simulink model "extractLocalMap"  (R2024a)
settings: Solver=FixedStepAuto  StartTime=0.0  StopTime=10.0  RelTol=1e-3
settings Model: Creator=cstabile  LastModifiedBy=cstabile
settings SFSimCC: SimTargetLang=C++

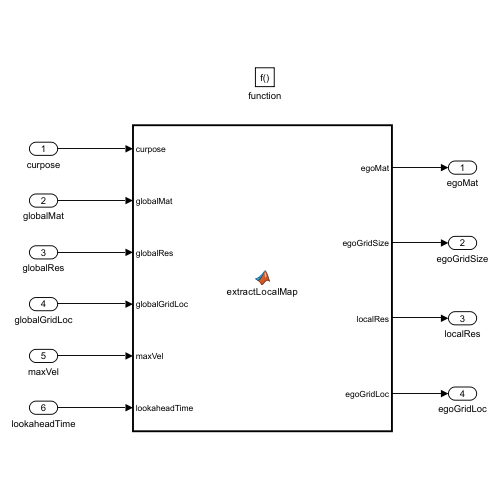
[thumbnail: Simulink's stored preview of the top-level diagram]
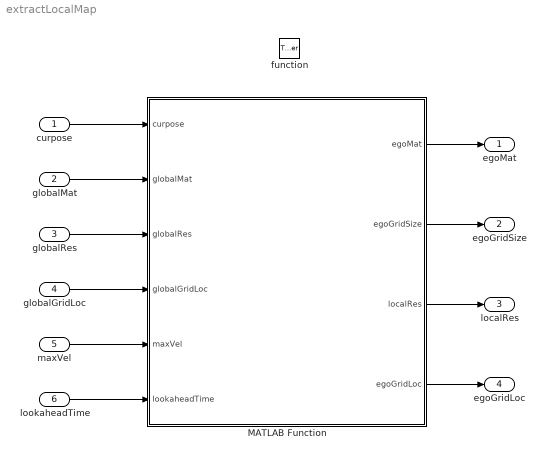
== system extractLocalMap ==
  curpose : Inport  PortDimensions=[1 3]
  globalMat : Inport  Port=2  OutDataTypeStr=boolean  PortDimensions=[1201 1201]
  globalRes : Inport  Port=3
  globalGridLoc : Inport  Port=4  PortDimensions=[1 2]
  maxVel : Inport  Port=5
  lookaheadTime : Inport  Port=6
  function : TriggerPort  TriggerType=function-call  VariantControl=(inherit)
  MATLAB Function : MATLAB Function  TreatAsAtomicUnit=on
  egoMat : Outport
  egoGridSize : Outport  Port=2
  localRes : Outport  Port=3
  egoGridLoc : Outport  Port=4
  wires:
  globalRes/1 -> MATLAB Function/3(globalRes)
  curpose/1 -> MATLAB Function/1(curpose)
  globalGridLoc/1 -> MATLAB Function/4(globalGridLoc)
  MATLAB Function/1(egoMat) -> egoMat/1
  globalMat/1 -> MATLAB Function/2(globalMat)
  maxVel/1 -> MATLAB Function/5(maxVel)
  lookaheadTime/1 -> MATLAB Function/6(lookaheadTime)
  MATLAB Function/2(egoGridSize) -> egoGridSize/1
  MATLAB Function/3(localRes) -> localRes/1
  MATLAB Function/4(egoGridLoc) -> egoGridLoc/1

== matlab function extractLocalMap/MATLAB Function ==
  data: curpose input; globalMat input; globalRes input; egoMat output size=[1201 1201]; egoGridSize output; localRes output; globalGridLoc input size=[1 2]; maxVel input; lookaheadTime input; egoGridLoc output size=[1 2]
function [egoMat,egoGridSize,localRes,egoGridLoc] = extractLocalMap(curpose,globalMat,globalRes,globalGridLoc,maxVel,lookaheadTime)
    persistent globalMap
    
    if isempty(globalMap)
        globalMap = binaryOccupancyMap(globalMat,globalRes);
        globalMap.GridLocationInWorld = globalGridLoc;
    else
        % Check if global map needs to be updated
        if ~isequal(globalMat,globalMap.occupancyMatrix)
            setOccupancy(globalMap,globalMat);
        end
        if ~isequal(globalGridLoc(1:2)',globalMap.GridLocationInWorld)
            globalMap.GridLocationInWorld = globalGridLoc;
        end
    end

    % Create and sync local map, then export occupancy matrix
    localRes = 1;
    mapSize = maxVel(1)*lookaheadTime*2;
    egoMap = binaryOccupancyMap(mapSize,mapSize,localRes);
    egoMap.LocalOriginInWorld = curpose(1:2);
    egoMap.GridOriginInLocal = -egoMap.GridSize/2/egoMap.Resolution;
    syncWith(egoMap,globalMap);

    % Extract region of interest
    egoGridSize = egoMap.GridSize;
    egoMat = occupancyMatrix(egoMap);
    egoGridLoc = zeros(1,2);
    egoGridLoc(1:2) = egoMap.GridLocationInWorld(1:2);
end
